simulink model "Aerodynamic_force_moment"  (R2018a)
settings: Solver=VariableStepAuto  StartTime=0.0  StopTime=10.0  RelTol=1e-3
settings Model: Creator=McQueen_Zero  LastModifiedBy=McQueen_Zero

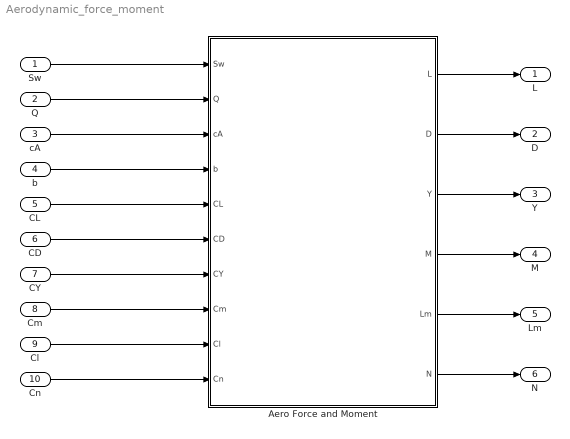
== system Aerodynamic_force_moment ==
  Sw : Inport
  Q : Inport  Port=2
  cA : Inport  Port=3
  b : Inport  Port=4
  CL : Inport  Port=5
  CD : Inport  Port=6
  CY : Inport  Port=7
  Cm : Inport  Port=8
  Cl : Inport  Port=9
  Cn : Inport  Port=10
  Aero Force and Moment : Subsystem
  L : Outport
  D : Outport  Port=2
  Y : Outport  Port=3
  M : Outport  Port=4
  Lm : Outport  Port=5
  N : Outport  Port=6
  wires:
  Sw/1 -> Aero Force and Moment/1(Sw)
  Q/1 -> Aero Force and Moment/2(Q)
  cA/1 -> Aero Force and Moment/3(cA)
  b/1 -> Aero Force and Moment/4(b)
  CL/1 -> Aero Force and Moment/5(CL)
  CD/1 -> Aero Force and Moment/6(CD)
  CY/1 -> Aero Force and Moment/7(CY)
  Cm/1 -> Aero Force and Moment/8(Cm)
  Cl/1 -> Aero Force and Moment/9(Cl)
  Cn/1 -> Aero Force and Moment/10(Cn)
  Aero Force and Moment/1(L) -> L/1
  Aero Force and Moment/2(D) -> D/1
  Aero Force and Moment/3(Y) -> Y/1
  Aero Force and Moment/4(M) -> M/1
  Aero Force and Moment/5(Lm) -> Lm/1
  Aero Force and Moment/6(N) -> N/1

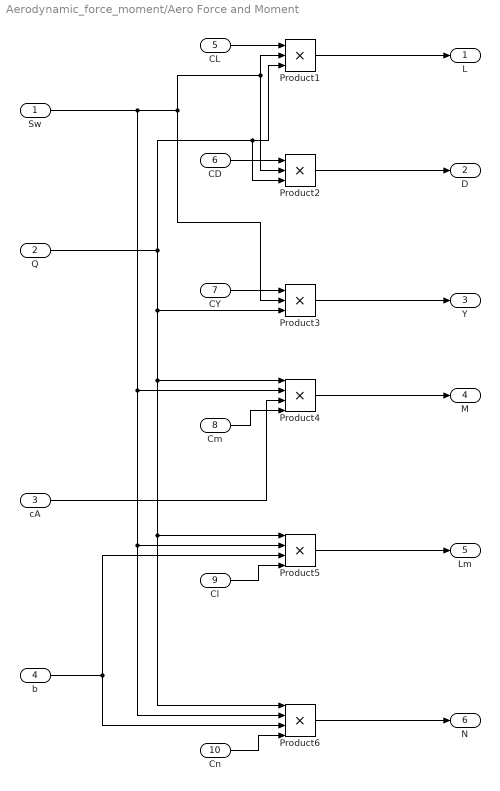
== system Aerodynamic_force_moment/Aero Force and Moment ==
  Sw : Inport
  Q : Inport  Port=2
  cA : Inport  Port=3
  b : Inport  Port=4
  CL : Inport  Port=5
  CD : Inport  Port=6
  CY : Inport  Port=7
  Cm : Inport  Port=8
  Cl : Inport  Port=9
  Cn : Inport  Port=10
  Product1 : Product  Inputs=3
  Product2 : Product  Inputs=3
  Product3 : Product  Inputs=3
  Product4 : Product  Inputs=4
  Product5 : Product  Inputs=4
  Product6 : Product  Inputs=4
  L : Outport
  D : Outport  Port=2
  Y : Outport  Port=3
  M : Outport  Port=4
  Lm : Outport  Port=5
  N : Outport  Port=6
  wires:
  Sw/1 -> Product4/2, Product5/2, Product6/2, Product3/2, Product1/2, Product2/2
  Q/1 -> Product2/3, Product1/3, Product6/1, Product5/1, Product4/1, Product3/3
  b/1 -> Product6/3, Product5/3
  Cn/1 -> Product6/4
  cA/1 -> Product4/3
  CL/1 -> Product1/1
  Cm/1 -> Product4/4
  Product4/1 -> M/1
  Product2/1 -> D/1
  CD/1 -> Product2/1
  Cl/1 -> Product5/4
  Product3/1 -> Y/1
  Product6/1 -> N/1
  Product5/1 -> Lm/1
  CY/1 -> Product3/1
  Product1/1 -> L/1
